simulink model "Fuel_Pump_V3_1_20201113_20KHz"  (R2019b)
settings: configuration reference "Configuration" (kept outside this file)
PreLoadFcn:
  | RTWConfigurationCB('preloadfcn', bdroot);
values from neighbouring files (symbols this model uses):
  MotorPara_Base_Frq = 666.0    [fuel_pump_V3_1_20201113_20kHz.sldd]
  MotorPara_Base_I = 50.0    [fuel_pump_V3_1_20201113_20kHz.sldd]
  MotorPara_Base_RPM = 12000.0    [fuel_pump_V3_1_20201113_20kHz.sldd]
  MotorPara_Base_V = 28.0    [fuel_pump_V3_1_20201113_20kHz.sldd]
  MotorPara_Ld = 1.287E-5    [fuel_pump_V3_1_20201113_20kHz.sldd]
  MotorPara_Lq = 2.052E-5    [fuel_pump_V3_1_20201113_20kHz.sldd]
  MotorPara_Ls = 8.3475E-5    [fuel_pump_V3_1_20201113_20kHz.sldd]
  MotorPara_P = 4.0    [fuel_pump_V3_1_20201113_20kHz.sldd]
  MotorPara_Rs = 0.01638    [fuel_pump_V3_1_20201113_20kHz.sldd]
  TPBRD_HALF = 1875.0    [fuel_pump_V3_1_20201113_20kHz.sldd]
  Ts_1kHz = 0.001    [fuel_pump_V3_1_20201113_20kHz.sldd]
  Ts_200Hz = 0.005    [fuel_pump_V3_1_20201113_20kHz.sldd]
  Ts_20KHz = 5.0E-5    [fuel_pump_V3_1_20201113_20kHz.sldd]
  Ts_40Hz = 0.025    [fuel_pump_V3_1_20201113_20kHz.sldd]
  Ts_50Hz = 0.02    [fuel_pump_V3_1_20201113_20kHz.sldd]
undefined symbols (not defined in the file or in its folder): DiscIntNeverNeededParam, Down, Up
libraries: c280xlib x22, c2833xlib x6, c2837xDlib x4, c28xdmclib x4, etargetslib x4, dspstat3 x2, c2000lib x1, idelinklib_common x1
(part 4 of 4)

== matlab function Fuel_Pump_V3_1_20201113_20KHz/CCP_Buffer/MATLAB Function ==
  data: Data_Buffer_ThetaSMO data_store_memory; Data_Buffer_ThetaAD2S data_store_memory; Data_Buffer_IqDem data_store_memory; Data_Buffer_IdDem data_store_memory; Data_Buffer_Id data_store_memory; Data_Buffer_Iq data_store_memory; Buffer_Flag data_store_memory; Buffer_Out_ThetaSMO data_store_memory; Buffer_Out_ThetaAD2S data_store_memory; Buffer_Out_IqDem data_store_memory; Buffer_Out_IdDem data_store_memory; Buffer_Out_Iq data_store_memory; Buffer_Out_Id data_store_memory
function Buffer_Reard
    global Data_Buffer_ThetaSMO Data_Buffer_ThetaAD2S;
    global Data_Buffer_IqDem    Data_Buffer_IdDem;
    global Data_Buffer_Iq       Data_Buffer_Id;
    global Buffer_Flag;
    
    global Buffer_Out_ThetaSMO Buffer_Out_ThetaAD2S;
    global Buffer_Out_IqDem    Buffer_Out_IdDem;
    global Buffer_Out_Iq       Buffer_Out_Id;
persistent count_out switch_count;

if isempty(count_out)
    count_out =single(1);
end
if isempty(switch_count)
    switch_count =single(1);
end

if(Buffer_Flag == 0)
    Buffer_Out_ThetaSMO  = single(-5);
    Buffer_Out_ThetaAD2S = single(-5);
    Buffer_Out_IqDem = single(-5);
    Buffer_Out_Iq    = single(-5);
    Buffer_Out_IdDem = single(-5);
    Buffer_Out_Id    = single(-5);
else
    if(count_out <= single(1000))
        switch switch_count
            case 1
                Buffer_Out_ThetaSMO  = Data_Buffer_ThetaSMO(count_out);
                switch_count = single(2);
            case 2
                Buffer_Out_ThetaAD2S = Data_Buffer_ThetaAD2S(count_out);
                switch_count = single(3);
            case 3
                Buffer_Out_IqDem = Data_Buffer_IqDem(count_out);
                switch_count = single(4);
            case 4
                Buffer_Out_Iq    = Data_Buffer_Iq(count_out);
                switch_count = single(5);
            case 5
                Buffer_Out_IdDem = Data_Buffer_IdDem(count_out);
                switch_count = single(6);
            case 6
                Buffer_Out_Id    = Data_Buffer_Id(count_out); 
                switch_count = single(1);
                count_out = count_out + single(1);
        end
    else
        Buffer_Out_ThetaSMO  = single(-5);
        Buffer_Out_ThetaAD2S = single(-5);
        Buffer_Out_IqDem = single(-5);
        Buffer_Out_Iq    = single(-5);
        Buffer_Out_IdDem = single(-5);
        Buffer_Out_Id    = single(-5);        
        count_out =single(1);
        Buffer_Flag = uint16(0);
    end
    
    
end
end

== matlab function Fuel_Pump_V3_1_20201113_20KHz/Motor_Control/Main Case /AD2S1210/If Action Subsystem/MATLAB Function ==
  data: Flag output
function Flag = Speed_Count
persistent AD2S_n_Count;
if isempty(AD2S_n_Count)
   AD2S_n_Count=uint16(1);
end
if(AD2S_n_Count > uint16(20))
    Flag = uint16(1);
    AD2S_n_Count = uint16(1);
else
    Flag = uint16(0);
	AD2S_n_Count = AD2S_n_Count + uint16(1);  
end
end

== matlab function Fuel_Pump_V3_1_20201113_20KHz/Motor_Control/Main Case /AD2S1210/If Action Subsystem/If Action Subsystem/MATLAB Function1 ==
  data: theta input; speed output single; theta_old input; Ts_20KHz parameter
function speed = Est_Speed(theta,theta_old, Ts_20KHz)

error = (theta - theta_old)*2*pi;
if(error > pi)
    error = error - 2*pi;
elseif(error <- pi)
	error = error + 2*pi;
end
speed = error/(Ts_20KHz*20)*30/pi;
% if(error>2*pi||error<-2*pi)
%     error = 0.0;
% end

end

== matlab function Fuel_Pump_V3_1_20201113_20KHz/Motor_Control/Main Case /AD2S1210/If Action Subsystem/MATLAB Function1 ==
  data: RAW_DATA input; Output output; RAW_DATA_OLD input; ControlMode input
function Output = AD2S1210_ERROR(RAW_DATA,RAW_DATA_OLD,ControlMode)
    if(abs(RAW_DATA - RAW_DATA_OLD) < uint16(1000))
        Output = uint16(RAW_DATA);
    elseif(abs(RAW_DATA - RAW_DATA_OLD) > uint16(63000))
        Output = uint16(RAW_DATA);
    else
        Output = uint16(RAW_DATA_OLD);
    end
    
    if(ControlMode == 0)
        Output = uint16(RAW_DATA);
    end
end

== matlab function Fuel_Pump_V3_1_20201113_20KHz/SCI_TX/SCI_TX/MATLAB Function ==
  data: High output; Low output; CPU_Timer data_store_memory
function [High,Low] = CPU_Timer
global CPU_Timer
    CPU_Timer = CPU_Timer + uint32(1);
    High = uint16(bitand(CPU_Timer,hex2dec('FFFF')));
    Low =uint16(bitand(CPU_Timer/(uint32(65535)),hex2dec('FFFF')));

end

== matlab function Fuel_Pump_V3_1_20201113_20KHz/SCI_TX/SCI_TX/MATLAB Function10 ==
  data: RAW_DATA input; TX_DATA output
function TX_DATA = SCI_Encoding_RPM(RAW_DATA)
LSB = single(1);
Real_Current = -single(RAW_DATA)/LSB;
if(Real_Current >= 0&&Real_Current<=20000)
    SCI_Buffer = uint16(Real_Current/single(1));
elseif(Real_Current>20000)
    SCI_Buffer = bitcmp(uint16(20000))+uint16(1);
else
    SCI_Buffer = uint16(0);
end
    TX_DATA = SCI_Buffer;
end

== matlab function Fuel_Pump_V3_1_20201113_20KHz/SCI_TX/SCI_TX/MATLAB Function23 ==
  data: TX_DATA input; TX_DATA_Hig output; TX_DATA_Low output
function [TX_DATA_Hig,TX_DATA_Low] = TransUint8(TX_DATA)
    TX_DATA_Low = uint8(bitshift(TX_DATA,-8));  %小端模式
    TX_DATA_Hig = uint8(bitand(TX_DATA,255));
end

== matlab function Fuel_Pump_V3_1_20201113_20KHz/SCI_TX/SCI_TX/MATLAB Function24 ==
  data: TX_DATA input; TX_DATA_Hig output; TX_DATA_Low output
function [TX_DATA_Hig,TX_DATA_Low] = TransUint8(TX_DATA)
    TX_DATA_Low = uint8(bitshift(TX_DATA,-8));  %小端模式
    TX_DATA_Hig = uint8(bitand(TX_DATA,255));
end

== matlab function Fuel_Pump_V3_1_20201113_20KHz/SCI_TX/FPM/MATLAB Function ==
  data: u input; y output
function y = FPM_checkLWFf(u)
persistent cnt;

if isempty(cnt)
    cnt = 0;
end

if((u >= -0.6) && (u <= 0.6))
    cnt = 0;
else
    cnt = cnt + 1;
end

if(cnt >= 3)
    y = uint16(1);
else
    y = uint16(0);
end
end

== matlab function Fuel_Pump_V3_1_20201113_20KHz/SCI_TX/FPM/MATLAB Function1 ==
  data: u input; y output
function y = FPM_checkResolver(u)
persistent cnt;

if isempty(cnt)
    cnt = 0;
end

if((u >= -12000) && (u <= 5))
    cnt = 0;
else
    cnt = cnt + 1;
end

if(cnt >= 3)
    y = uint16(1);
else
    y = uint16(0);
end
end

== matlab function Fuel_Pump_V3_1_20201113_20KHz/SCI_TX/FPM/MATLAB Function2 ==
  data: MOST1 input; y output; MOST2 input
function y = FPM_checkMOSTSensor(MOST1,MOST2)
persistent cnt1;
persistent cnt2;
if isempty(cnt1)
    cnt1 = 0;
end
if isempty(cnt2)
    cnt2 = 0;
end

if(MOST1 <= 180)
    cnt1 = 0;
else
    cnt1 = cnt1 + 1;
end

if(MOST2 <= 180)
    cnt2 = 0;
else
    cnt2 = cnt2 + 1;
end

if((cnt1 >= 3) || (cnt2 >= 3))
    y = uint16(1);
else
    y = uint16(0);
end
end

== matlab function Fuel_Pump_V3_1_20201113_20KHz/SCI_TX/FPM/MATLAB Function3 ==
  data: u input; y output
function y = FPM_checkWindingUTSensor(u)
persistent cnt;

if isempty(cnt)
    cnt = 0;
end

if((u >= -180) && (u <= 180))
    cnt = 0;
else
    cnt = cnt + 1;
end

if(cnt >= 3)
    y = uint16(1);
else
    y = uint16(0);
end
end

== matlab function Fuel_Pump_V3_1_20201113_20KHz/SCI_TX/FPM/MATLAB Function4 ==
  data: u input; y output
function y = FPM_checkWindingVTSensor(u)
persistent cnt;

if isempty(cnt)
    cnt = 0;
end

if((u >= -180) && (u <= 180))
    cnt = 0;
else
    cnt = cnt + 1;
end

if(cnt >= 3)
    y = uint16(1);
else
    y = uint16(0);
end
end

== matlab function Fuel_Pump_V3_1_20201113_20KHz/SCI_TX/FPM/MATLAB Function5 ==
  data: UI input; y output; VI input; WI input
function y = FPM_checkWindingISensor(UI,VI,WI)
persistent cnt_UI;
persistent cnt_VI;
persistent cnt_WI;

if isempty(cnt_UI)
    cnt_UI = 0;
end

if isempty(cnt_VI)
    cnt_VI = 0;
end

if isempty(cnt_WI)
    cnt_WI = 0;
end

if((UI >= -1.5) && (UI <= 1.5))
    cnt_UI = 0;
else
    cnt_UI = cnt_UI + 1;
end

if((VI >= -1.5) && (VI <= 1.5))
    cnt_VI = 0;
else
    cnt_VI = cnt_VI + 1;
end

if((WI >= -1.5) && (WI <= 1.5))
    cnt_WI = 0;
else
    cnt_WI = cnt_WI + 1;
end


if((cnt_UI >= 3) || (cnt_VI >= 3) || (cnt_WI >= 3))
    y = uint16(1);
else
    y = uint16(0);
end
end

== matlab function Fuel_Pump_V3_1_20201113_20KHz/SCI_TX/FPM/MATLAB Function6 ==
  data: u input; y output
function y = FPM_checkOvrLimWindingI(u)

if(u == 0)
    y = uint16(0);
else
    y = uint16(1);
end

end

== matlab function Fuel_Pump_V3_1_20201113_20KHz/SCI_TX/FPM/MATLAB Function7 ==
  data: T1 input; y output; T2 input; bFlt_OvrLim_TempMOST data_store_memory
function y = FPM_checkOvrLimMOST(T1,T2)
global bFlt_OvrLim_TempMOST;
persistent cnt1;
persistent cnt2;
if isempty(cnt1)
    cnt1 = 0;
end
if isempty(cnt2)
    cnt2 = 0;
end

if(T1 <= 90)
    cnt1 = 0;
else
    cnt1 = cnt1 + 1;
end

if(T2 <= 120)
    cnt2 = 0;
else
    cnt2 = cnt2 + 1;
end

if((cnt1 >= 12) || (cnt2 >= 12))
    bFlt_OvrLim_TempMOST = uint16(1);
end
    y = bFlt_OvrLim_TempMOST;
end

== matlab function Fuel_Pump_V3_1_20201113_20KHz/SCI_TX/FPM/MATLAB Function8 ==
  data: T input; y output; bFlt_OvrLim_TempUT data_store_memory
function y = FPM_checkOvrLimWindingUT(T)
global bFlt_OvrLim_TempUT;
persistent cnt1;
if isempty(cnt1)
    cnt1 = 0;
end


if(T <= 120)
    cnt1 = 0;
else
    cnt1 = cnt1 + 1;
end



if(cnt1 >= 12)
    bFlt_OvrLim_TempUT = uint16(1);
end
    y = bFlt_OvrLim_TempUT;
end

== matlab function Fuel_Pump_V3_1_20201113_20KHz/SCI_TX/FPM/MATLAB Function9 ==
  data: T input; y output; bFlt_OvrLim_TempVT data_store_memory
function y = FPM_checkOvrLimWindingVT(T)
global bFlt_OvrLim_TempVT;
persistent cnt1;
if isempty(cnt1)
    cnt1 = 0;
end


if(T <= 120)
    cnt1 = 0;
else
    cnt1 = cnt1 + 1;
end



if(cnt1 >= 12)
    bFlt_OvrLim_TempVT = uint16(1);
end
    y = bFlt_OvrLim_TempVT;
end

== matlab function Fuel_Pump_V3_1_20201113_20KHz/SCI_TX/SCI_TX/MATLAB Function25 ==
  data: TX_DATA input; TX_DATA_Hig output; TX_DATA_Low output
function [TX_DATA_Hig,TX_DATA_Low] = TransUint8(TX_DATA)
    TX_DATA_Low = uint8(bitshift(TX_DATA,-8));  %小端模式
    TX_DATA_Hig = uint8(bitand(TX_DATA,255));
end

== matlab function Fuel_Pump_V3_1_20201113_20KHz/SCI_TX/SCI_TX/MATLAB Function1 ==
  data: RAW_DATA input; TX_DATA output
function TX_DATA = SCI_Encoding_RPM(RAW_DATA)
LSB = single(1);
Real_Current = -single(RAW_DATA)/LSB;
if(Real_Current >= 0&&Real_Current<=20000)
    SCI_Buffer = uint16(Real_Current/single(1));
elseif(Real_Current>20000)
    SCI_Buffer = bitcmp(uint16(20000))+uint16(1);
else
    SCI_Buffer = uint16(0);
end
    TX_DATA = SCI_Buffer;
end

== matlab function Fuel_Pump_V3_1_20201113_20KHz/SCI_TX/SCI_TX/MATLAB Function26 ==
  data: TX_DATA input; TX_DATA_Hig output; TX_DATA_Low output
function [TX_DATA_Hig,TX_DATA_Low] = TransUint8(TX_DATA)
    TX_DATA_Low = uint8(bitshift(TX_DATA,-8));  %小端模式
    TX_DATA_Hig = uint8(bitand(TX_DATA,255));
end

== matlab function Fuel_Pump_V3_1_20201113_20KHz/SCI_TX/SCI_TX/MATLAB Function11 ==
  data: RAW_DATA input; TX_DATA output
function TX_DATA = SCI_Encoding_LWF(RAW_DATA)
LSB = single(16/32767);
Real_DATA = single(RAW_DATA)/LSB;
if(Real_DATA >= 0&&Real_DATA<=32767)
    SCI_Buffer = uint16(Real_DATA/single(1));
elseif(Real_DATA>32767)
    SCI_Buffer = uint16(32767);
else
    SCI_Buffer = uint16(0);
end
    TX_DATA = SCI_Buffer;
end

== matlab function Fuel_Pump_V3_1_20201113_20KHz/SCI_TX/SCI_TX/MATLAB Function12 ==
  data: RAW_DATA input; TX_DATA output
function TX_DATA = SCI_Encoding_LWF(RAW_DATA)
LSB = single(16/32767);
Real_DATA = single(RAW_DATA)/LSB;
if(Real_DATA >= 0&&Real_DATA<=32767)
    SCI_Buffer = uint16(Real_DATA/single(1));
elseif(Real_DATA>32767)
    SCI_Buffer = uint16(32767);
else
    SCI_Buffer = uint16(0);
end
    TX_DATA = SCI_Buffer;
end

== matlab function Fuel_Pump_V3_1_20201113_20KHz/SCI_TX/SCI_TX/MATLAB Function13 ==
  data: RAW_DATA input; TX_DATA output
function TX_DATA = SCI_Encoding_LWF(RAW_DATA)
LSB = single(16/32767);
Real_DATA = single(RAW_DATA)/LSB;
if(Real_DATA >= 0&&Real_DATA<=32767)
    SCI_Buffer = uint16(Real_DATA/single(1));
elseif(Real_DATA>32767)
    SCI_Buffer = uint16(32767);
else
    SCI_Buffer = uint16(0);
end
    TX_DATA = SCI_Buffer;
end

== matlab function Fuel_Pump_V3_1_20201113_20KHz/SCI_TX/SCI_TX/MATLAB Function14 ==
  data: RAW_DATA input; TX_DATA output
function TX_DATA = SCI_Encoding_Temp(RAW_DATA)
LSB = single(1/100);
Real_Current = single(RAW_DATA)/LSB;
if(Real_Current >= 0&&Real_Current<=25600)
    SCI_Buffer = uint16(Real_Current/single(1));
elseif(Real_Current>25600)
    SCI_Buffer = uint16(25600);
elseif(Real_Current < 0&&Real_Current>=-25600)
    SCI_Buffer = bitcmp(uint16(Real_Current/single(-1)))+uint16(1);
else
    SCI_Buffer = bitcmp(uint16(25600))+uint16(1);
end
    TX_DATA = SCI_Buffer;
end

== matlab function Fuel_Pump_V3_1_20201113_20KHz/SCI_TX/SCI_TX/MATLAB Function15 ==
  data: RAW_DATA input; TX_DATA output
function TX_DATA = SCI_Encoding_Temp(RAW_DATA)
LSB = single(1/100);
Real_Current = single(RAW_DATA)/LSB;
if(Real_Current >= 0&&Real_Current<=25600)
    SCI_Buffer = uint16(Real_Current/single(1));
elseif(Real_Current>25600)
    SCI_Buffer = uint16(25600);
elseif(Real_Current < 0&&Real_Current>=-25600)
    SCI_Buffer = bitcmp(uint16(Real_Current/single(-1)))+uint16(1);
else
    SCI_Buffer = bitcmp(uint16(25600))+uint16(1);
end
    TX_DATA = SCI_Buffer;
end

== matlab function Fuel_Pump_V3_1_20201113_20KHz/SCI_TX/SCI_TX/MATLAB Function16 ==
  data: RAW_DATA input; TX_DATA output
function TX_DATA = SCI_Encoding_Temp(RAW_DATA)
LSB = single(1/100);
Real_Current = single(RAW_DATA)/LSB;
if(Real_Current >= 0&&Real_Current<=25600)
    SCI_Buffer = uint16(Real_Current/single(1));
elseif(Real_Current>25600)
    SCI_Buffer = uint16(25600);
elseif(Real_Current < 0&&Real_Current>=-25600)
    SCI_Buffer = bitcmp(uint16(Real_Current/single(-1)))+uint16(1);
else
    SCI_Buffer = bitcmp(uint16(25600))+uint16(1);
end
    TX_DATA = SCI_Buffer;
end

== matlab function Fuel_Pump_V3_1_20201113_20KHz/SCI_TX/SCI_TX/MATLAB Function17 ==
  data: RAW_DATA input; TX_DATA output
function TX_DATA = SCI_Encoding_Temp(RAW_DATA)
LSB = single(1/100);
Real_Current = single(RAW_DATA)/LSB;
if(Real_Current >= 0&&Real_Current<=25600)
    SCI_Buffer = uint16(Real_Current/single(1));
elseif(Real_Current>25600)
    SCI_Buffer = uint16(25600);
elseif(Real_Current < 0&&Real_Current>=-25600)
    SCI_Buffer = bitcmp(uint16(Real_Current/single(-1)))+uint16(1);
else
    SCI_Buffer = bitcmp(uint16(25600))+uint16(1);
end
    TX_DATA = SCI_Buffer;
end

== matlab function Fuel_Pump_V3_1_20201113_20KHz/SCI_TX/SCI_TX/MATLAB Function18 ==
  data: RAW_DATA input; TX_DATA output
function TX_DATA = SCI_Encoding_WFmf(RAW_DATA)
LSB = single(500/32767);
Real_DATA = single(RAW_DATA)/LSB;
if(Real_DATA >= 0&&Real_DATA<=32767)
    SCI_Buffer = uint16(Real_DATA/single(1));
elseif(Real_DATA>32767)
    SCI_Buffer = uint16(32767);
else
    SCI_Buffer = uint16(0);
end
    TX_DATA = SCI_Buffer;
end

== matlab function Fuel_Pump_V3_1_20201113_20KHz/SCI_TX/SCI_TX/MATLAB Function19 ==
  data: RAW_DATA input; TX_DATA output
function TX_DATA = SCI_Encoding_Res(RAW_DATA)
LSB = single(2*pi/32767);
Real_DATA = single(single(RAW_DATA)/single(65535)*single(2*pi))/LSB;
if(Real_DATA >= 0&&Real_DATA<=32767)
    SCI_Buffer = uint16(Real_DATA/single(1));
elseif(Real_DATA>32767)
    SCI_Buffer = uint16(32767);
else
    SCI_Buffer = uint16(0);
end
    TX_DATA = SCI_Buffer;
end

== matlab function Fuel_Pump_V3_1_20201113_20KHz/SCI_TX/SCI_TX/MATLAB Function2 ==
  data: RAW_DATA input; TX_DATA output
function TX_DATA = SCI_Encoding_Current(RAW_DATA)
LSB = single(1/100);
Real_Current = single(RAW_DATA)*single(100)/LSB;
if(Real_Current >= 0&&Real_Current<=25600)
    SCI_Buffer = uint16(Real_Current/single(1));
elseif(Real_Current>25600)
    SCI_Buffer = uint16(25600);
elseif(Real_Current < 0&&Real_Current>=-25600)
    SCI_Buffer = bitcmp(uint16(Real_Current/single(-1)))+uint16(1);
else
    SCI_Buffer = bitcmp(uint16(25600))+uint16(1);
end
    TX_DATA = SCI_Buffer;
end

== matlab function Fuel_Pump_V3_1_20201113_20KHz/SCI_TX/SCI_TX/MATLAB Function21 ==
  data: U1 input; U2 input; U3 input; U4 input; U5 input; U6 input; U7 input; U8 input; U9 input; U10 input; U11 input; EFP2 output
function EFP2 = PackEFP2(U1,U2,U3,U4,U5,U6,U7,U8,U9,U10,U11)

D0 = uint16((1 == U1));
D1 = uint16((1 == U2));
D2 = uint16((1 == U3));
D3 = uint16((1 == U4));
D4 = uint16((1 == U5));
D5 = uint16((1 == U6));
D6 = uint16((1 == U7));
D7 = uint16((1 == U8));
D8 = uint16((1 == U9));
D9 = uint16((1 == U10));
D10 = uint16((1 == U11));

EFP2 = (bitshift(D0,0) + bitshift(D1,1) + bitshift(D2,2) + bitshift(D3,3)  + bitshift(D4,4) + bitshift(D5,5) + bitshift(D6,6) + bitshift(D7,7) + bitshift(D8,8) + bitshift(D9,9) + bitshift(D10,10));
end

== matlab function Fuel_Pump_V3_1_20201113_20KHz/SCI_TX/SCI_TX/MATLAB Function22 ==
  data: u input; TX_DATA output
function TX_DATA = Sumsrc(u)

TX_DATA = uint8(bitand(sum(u(4:50)),255));
end

== matlab function Fuel_Pump_V3_1_20201113_20KHz/SCI_TX/SCI_TX/MATLAB Function27 ==
  data: TX_DATA input; TX_DATA_Hig output; TX_DATA_Low output
function [TX_DATA_Hig,TX_DATA_Low] = TransUint8(TX_DATA)
    TX_DATA_Low = uint8(bitshift(TX_DATA,-8));  %小端模式
    TX_DATA_Hig = uint8(bitand(TX_DATA,255));
end

== matlab function Fuel_Pump_V3_1_20201113_20KHz/SCI_TX/SCI_TX/MATLAB Function28 ==
  data: TX_DATA input; TX_DATA_Hig output; TX_DATA_Low output
function [TX_DATA_Hig,TX_DATA_Low] = TransUint8(TX_DATA)
    TX_DATA_Low = uint8(bitshift(TX_DATA,-8));  %小端模式
    TX_DATA_Hig = uint8(bitand(TX_DATA,255));
end

== matlab function Fuel_Pump_V3_1_20201113_20KHz/SCI_TX/SCI_TX/MATLAB Function29 ==
  data: TX_DATA input; TX_DATA_Hig output; TX_DATA_Low output
function [TX_DATA_Hig,TX_DATA_Low] = TransUint8(TX_DATA)
    TX_DATA_Low = uint8(bitshift(TX_DATA,-8));  %小端模式
    TX_DATA_Hig = uint8(bitand(TX_DATA,255));
end

== matlab function Fuel_Pump_V3_1_20201113_20KHz/SCI_TX/SCI_TX/MATLAB Function3 ==
  data: RAW_DATA input; TX_DATA output
function TX_DATA = SCI_Encoding_Current(RAW_DATA)
LSB = single(1/100);
Real_Current = single(RAW_DATA)*single(100)/LSB;
if(Real_Current >= 0&&Real_Current<=25600)
    SCI_Buffer = uint16(Real_Current/single(1));
elseif(Real_Current>25600)
    SCI_Buffer = uint16(25600);
elseif(Real_Current < 0&&Real_Current>=-25600)
    SCI_Buffer = bitcmp(uint16(Real_Current/single(-1)))+uint16(1);
else
    SCI_Buffer = bitcmp(uint16(25600))+uint16(1);
end
    TX_DATA =SCI_Buffer;
end

== matlab function Fuel_Pump_V3_1_20201113_20KHz/SCI_TX/SCI_TX/MATLAB Function30 ==
  data: TX_DATA input; TX_DATA_Hig output; TX_DATA_Low output
function [TX_DATA_Hig,TX_DATA_Low] = TransUint8(TX_DATA)
    TX_DATA_Low = uint8(bitshift(TX_DATA,-8));  %小端模式
    TX_DATA_Hig = uint8(bitand(TX_DATA,255));
end

== matlab function Fuel_Pump_V3_1_20201113_20KHz/SCI_TX/SCI_TX/MATLAB Function31 ==
  data: TX_DATA input; TX_DATA_Hig output; TX_DATA_Low output
function [TX_DATA_Hig,TX_DATA_Low] = TransUint8(TX_DATA)
    TX_DATA_Low = uint8(bitshift(TX_DATA,-8));  %小端模式
    TX_DATA_Hig = uint8(bitand(TX_DATA,255));
end

== matlab function Fuel_Pump_V3_1_20201113_20KHz/SCI_TX/SCI_TX/MATLAB Function32 ==
  data: TX_DATA input; TX_DATA_Hig output; TX_DATA_Low output
function [TX_DATA_Hig,TX_DATA_Low] = TransUint8(TX_DATA)
    TX_DATA_Low = uint8(bitshift(TX_DATA,-8));  %小端模式
    TX_DATA_Hig = uint8(bitand(TX_DATA,255));
end

== matlab function Fuel_Pump_V3_1_20201113_20KHz/SCI_TX/SCI_TX/MATLAB Function33 ==
  data: TX_DATA input; TX_DATA_Hig output; TX_DATA_Low output
function [TX_DATA_Hig,TX_DATA_Low] = TransUint8(TX_DATA)
    TX_DATA_Low = uint8(bitshift(TX_DATA,-8));  %小端模式
    TX_DATA_Hig = uint8(bitand(TX_DATA,255));
end

== matlab function Fuel_Pump_V3_1_20201113_20KHz/SCI_TX/SCI_TX/MATLAB Function34 ==
  data: TX_DATA input; TX_DATA_Hig output; TX_DATA_Low output
function [TX_DATA_Hig,TX_DATA_Low] = TransUint8(TX_DATA)
    TX_DATA_Low = uint8(bitshift(TX_DATA,-8));  %小端模式
    TX_DATA_Hig = uint8(bitand(TX_DATA,255));
end

== matlab function Fuel_Pump_V3_1_20201113_20KHz/SCI_TX/SCI_TX/MATLAB Function35 ==
  data: TX_DATA input; TX_DATA_Hig output; TX_DATA_Low output
function [TX_DATA_Hig,TX_DATA_Low] = TransUint8(TX_DATA)
    TX_DATA_Low = uint8(bitshift(TX_DATA,-8));  %小端模式
    TX_DATA_Hig = uint8(bitand(TX_DATA,255));
end

== matlab function Fuel_Pump_V3_1_20201113_20KHz/SCI_TX/SCI_TX/MATLAB Function36 ==
  data: TX_DATA input; TX_DATA_Hig output; TX_DATA_Low output
function [TX_DATA_Hig,TX_DATA_Low] = TransUint8(TX_DATA)
    TX_DATA_Low = uint8(bitshift(TX_DATA,-8));  %小端模式
    TX_DATA_Hig = uint8(bitand(TX_DATA,255));
end

== matlab function Fuel_Pump_V3_1_20201113_20KHz/SCI_TX/SCI_TX/MATLAB Function37 ==
  data: TX_DATA input; TX_DATA_Hig output; TX_DATA_Low output
function [TX_DATA_Hig,TX_DATA_Low] = TransUint8(TX_DATA)
    TX_DATA_Low = uint8(bitshift(TX_DATA,-8));  %小端模式
    TX_DATA_Hig = uint8(bitand(TX_DATA,255));
end

== matlab function Fuel_Pump_V3_1_20201113_20KHz/SCI_TX/SCI_TX/MATLAB Function38 ==
  data: TX_DATA input; TX_DATA_Hig output; TX_DATA_Low output
function [TX_DATA_Hig,TX_DATA_Low] = TransUint8(TX_DATA)
    TX_DATA_Low = uint8(bitshift(TX_DATA,-8));  %小端模式
    TX_DATA_Hig = uint8(bitand(TX_DATA,255));
end

== matlab function Fuel_Pump_V3_1_20201113_20KHz/SCI_TX/SCI_TX/MATLAB Function39 ==
  data: TX_DATA input; TX_DATA_Hig output; TX_DATA_Low output
function [TX_DATA_Hig,TX_DATA_Low] = TransUint8(TX_DATA)
    TX_DATA_Low = uint8(bitshift(TX_DATA,-8));  %小端模式
    TX_DATA_Hig = uint8(bitand(TX_DATA,255));
end

== matlab function Fuel_Pump_V3_1_20201113_20KHz/SCI_TX/SCI_TX/MATLAB Function4 ==
  data: TX_DATA input; TX_DATA_Hig output; TX_DATA_Low output
function [TX_DATA_Hig,TX_DATA_Low] = TransUint8(TX_DATA)
    TX_DATA_Low = uint8(bitshift(TX_DATA,-8));  %小端模式
    TX_DATA_Hig = uint8(bitand(TX_DATA,255));
end

== matlab function Fuel_Pump_V3_1_20201113_20KHz/SCI_TX/SCI_TX/MATLAB Function40 ==
  data: TX_DATA input; TX_DATA_Hig output; TX_DATA_Low output
function [TX_DATA_Hig,TX_DATA_Low] = TransUint8(TX_DATA)
    TX_DATA_Low = uint8(bitshift(TX_DATA,-8));  %小端模式
    TX_DATA_Hig = uint8(bitand(TX_DATA,255));
end

== matlab function Fuel_Pump_V3_1_20201113_20KHz/SCI_TX/SCI_TX/MATLAB Function41 ==
  data: TX_DATA input; TX_DATA_Hig output; TX_DATA_Low output
function [TX_DATA_Hig,TX_DATA_Low] = TransUint8(TX_DATA)
    TX_DATA_Low = uint8(bitshift(TX_DATA,-8));  %小端模式
    TX_DATA_Hig = uint8(bitand(TX_DATA,255));
end

== matlab function Fuel_Pump_V3_1_20201113_20KHz/SCI_TX/SCI_TX/MATLAB Function42 ==
  data: TX_DATA input; TX_DATA_Hig output; TX_DATA_Low output
function [TX_DATA_Hig,TX_DATA_Low] = TransUint8(TX_DATA)
    TX_DATA_Low = uint8(bitshift(TX_DATA,-8));  %小端模式
    TX_DATA_Hig = uint8(bitand(TX_DATA,255));
end

== matlab function Fuel_Pump_V3_1_20201113_20KHz/SCI_TX/SCI_TX/MATLAB Function43 ==
  data: TX_DATA input; TX_DATA_Hig output; TX_DATA_Low output
function [TX_DATA_Hig,TX_DATA_Low] = TransUint8(TX_DATA)
    TX_DATA_Low = uint8(bitshift(TX_DATA,-8));  %小端模式
    TX_DATA_Hig = uint8(bitand(TX_DATA,255));
end

== matlab function Fuel_Pump_V3_1_20201113_20KHz/SCI_TX/SCI_TX/MATLAB Function44 ==
  data: TX_DATA input; TX_DATA_Hig output; TX_DATA_Low output
function [TX_DATA_Hig,TX_DATA_Low] = TransUint8(TX_DATA)
    TX_DATA_Low = uint8(bitshift(TX_DATA,-8));  %小端模式
    TX_DATA_Hig = uint8(bitand(TX_DATA,255));
end

== matlab function Fuel_Pump_V3_1_20201113_20KHz/SCI_TX/SCI_TX/MATLAB Function5 ==
  data: RAW_DATA input; TX_DATA output
function TX_DATA = SCI_Encoding_Current(RAW_DATA)
LSB = single(1/100);
Real_Current = single(RAW_DATA)*single(100)/LSB;
if(Real_Current >= 0&&Real_Current<=25600)
    SCI_Buffer = uint16(Real_Current/single(1));
elseif(Real_Current>25600)
    SCI_Buffer = uint16(25600);
elseif(Real_Current < 0&&Real_Current>=-25600)
    SCI_Buffer = bitcmp(uint16(Real_Current/single(-1)))+uint16(1);
else
    SCI_Buffer = bitcmp(uint16(25600))+uint16(1);
end
    TX_DATA = SCI_Buffer;
end

== matlab function Fuel_Pump_V3_1_20201113_20KHz/SCI_TX/SCI_TX/MATLAB Function6 ==
  data: RAW_DATA input; TX_DATA output
function TX_DATA = SCI_Encoding_Current(RAW_DATA)
LSB = single(1/100);
Real_Current = single(RAW_DATA)*single(100)/LSB;
if(Real_Current >= 0&&Real_Current<=25600)
    SCI_Buffer = uint16(Real_Current/single(1));
elseif(Real_Current>25600)
    SCI_Buffer = uint16(25600);
elseif(Real_Current < 0&&Real_Current>=-25600)
    SCI_Buffer = bitcmp(uint16(Real_Current/single(-1)))+uint16(1);
else
    SCI_Buffer = bitcmp(uint16(25600))+uint16(1);
end
    TX_DATA = SCI_Buffer;
end

== matlab function Fuel_Pump_V3_1_20201113_20KHz/SCI_TX/SCI_TX/MATLAB Function7 ==
  data: RAW_DATA input; TX_DATA output
function TX_DATA = SCI_Encoding_Current(RAW_DATA)
LSB = single(1/100);
Real_Current = single(RAW_DATA)*single(100)/LSB;
if(Real_Current >= 0&&Real_Current<=25600)
    SCI_Buffer = uint16(Real_Current/single(1));
elseif(Real_Current>25600)
    SCI_Buffer = uint16(25600);
elseif(Real_Current < 0&&Real_Current>=-25600)
    SCI_Buffer = bitcmp(uint16(Real_Current/single(-1)))+uint16(1);
else
    SCI_Buffer = bitcmp(uint16(25600))+uint16(1);
end
    TX_DATA = SCI_Buffer;
end

== matlab function Fuel_Pump_V3_1_20201113_20KHz/SCI_TX/SCI_TX/MATLAB Function8 ==
  data: RAW_DATA input; TX_DATA output
function TX_DATA = SCI_Encoding_Current(RAW_DATA)
LSB = single(1/100);
Real_Current = single(RAW_DATA)*single(100)/LSB;
if(Real_Current >= 0&&Real_Current<=25600)
    SCI_Buffer = uint16(Real_Current/single(1));
elseif(Real_Current>25600)
    SCI_Buffer = uint16(25600);
elseif(Real_Current < 0&&Real_Current>=-25600)
    SCI_Buffer = bitcmp(uint16(Real_Current/single(-1)))+uint16(1);
else
    SCI_Buffer = bitcmp(uint16(25600))+uint16(1);
end
    TX_DATA = SCI_Buffer;
end

== matlab function Fuel_Pump_V3_1_20201113_20KHz/SCI_TX/SCI_TX/MATLAB Function9 ==
  data: RAW_DATA input; TX_DATA output
function TX_DATA = SCI_Encoding_Current(RAW_DATA)
LSB = single(1/100);
Real_Current = single(RAW_DATA)*single(100)/LSB;
if(Real_Current >= 0&&Real_Current<=25600)
    SCI_Buffer = uint16(Real_Current/single(1));
elseif(Real_Current>25600)
    SCI_Buffer = uint16(25600);
elseif(Real_Current < 0&&Real_Current>=-25600)
    SCI_Buffer = bitcmp(uint16(Real_Current/single(-1)))+uint16(1);
else
    SCI_Buffer = bitcmp(uint16(25600))+uint16(1);
end
    TX_DATA = SCI_Buffer;
end
